simulink model "tp1"  (R2019a)
settings: Solver=VariableStepAuto  StartTime=0.0  StopTime=15  FixedStep=0.05  RelTol=1e-3
undefined symbols (not defined in the file): g, l, x0
settings Model: Creator=tsadurni  LastModifiedBy=tsadurni

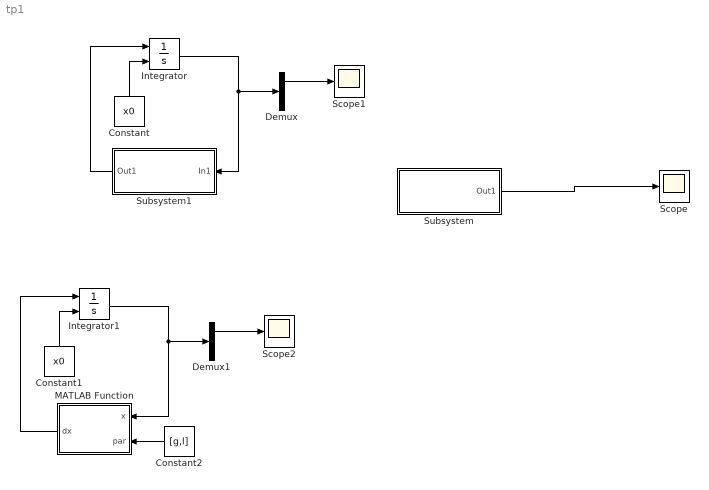
== system tp1 ==
  Constant : Constant  Value=x0
  Constant1 : Constant  Value=x0
  Constant2 : Constant  Value=[g,l]
  Demux : Demux  Outputs=2
  Demux1 : Demux  Outputs=2
  Integrator : Integrator  InitialConditionSource=external
  Integrator1 : Integrator  InitialConditionSource=external
  MATLAB Function : MATLAB Function  TreatAsAtomicUnit=on
  Scope : Scope
  Scope1 : Scope
  Scope2 : Scope
  Subsystem : Subsystem
  Subsystem1 : Subsystem
  wires:
  Subsystem/1(Out1) -> Scope/1
  Constant/1 -> Integrator/2
  Subsystem1/1(Out1) -> Integrator/1
  Integrator/1 -> Subsystem1/1(In1), Demux/1
  Demux/1 -> Scope1/1
  Integrator1/1 -> MATLAB Function/1(x), Demux1/1
  Constant1/1 -> Integrator1/2
  MATLAB Function/1(dx) -> Integrator1/1
  Demux1/1 -> Scope2/1
  Constant2/1 -> MATLAB Function/2(par)

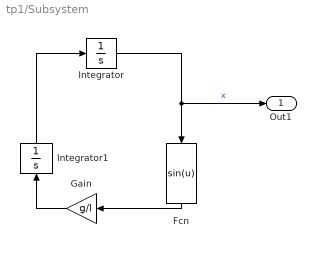
== system tp1/Subsystem ==
  Fcn : Fcn  Expr=sin(u)
  Gain : Gain  Gain=g/l
  Integrator : Integrator
  Integrator1 : Integrator  InitialCondition=0.05
  Out1 : Outport
  wires:
  Integrator/1 -> Out1/1, Fcn/1  "x"
  Fcn/1 -> Gain/1
  Integrator1/1 -> Integrator/1
  Gain/1 -> Integrator1/1

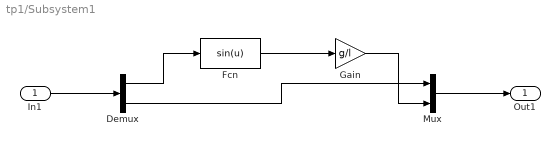
== system tp1/Subsystem1 ==
  In1 : Inport
  Demux : Demux  Outputs=2
  Fcn : Fcn  Expr=sin(u)
  Gain : Gain  Gain=g/l
  Mux : Mux  Inputs=2
  Out1 : Outport
  wires:
  In1/1 -> Demux/1
  Mux/1 -> Out1/1
  Fcn/1 -> Gain/1
  Demux/1 -> Fcn/1
  Gain/1 -> Mux/2
  Demux/2 -> Mux/1

== matlab function tp1/MATLAB Function ==
  data: x input; dx output; par input
function dx = fcn(x,par)

dx = [x(2); par(1)/par(2)*sin(x(1))]
